simulink model "ASMod_VolEff"  (R2016b)
settings: configuration reference "CodeGenConfigSet" (kept outside this file)
values from neighbouring files (symbols this model uses):
  ASMod_facEGRCor_MAP = Calibration.Parameter    [init_ASMod_VolEff.m]    (also in init_ASMod_VolEff_SIL.m = Simulink.Parameter)
  ASMod_facEGRCor_MAPX = Calibration.Parameter    [init_ASMod_VolEff.m]    (also in init_ASMod_VolEff_SIL.m = Simulink.Parameter)
  ASMod_facEGRCor_MAPY = Calibration.Parameter    [init_ASMod_VolEff.m]    (also in init_ASMod_VolEff_SIL.m = Simulink.Parameter)
  ASMod_facIntMnfDsTempCor_C = Calibration.Parameter    [init_ASMod_VolEff.m]    (also in init_ASMod_VolEff_SIL.m = Simulink.Parameter)
  ASMod_facVolEffBas_MAP = Calibration.Parameter    [init_ASMod_VolEff.m]    (also in init_ASMod_VolEff_SIL.m = Simulink.Parameter)
  ASMod_facVolEffBas_MAPX = Calibration.Parameter    [init_ASMod_VolEff.m]    (also in init_ASMod_VolEff_SIL.m = Simulink.Parameter)
  ASMod_facVolEffBas_MAPY = Calibration.Parameter    [init_ASMod_VolEff.m]    (also in init_ASMod_VolEff_SIL.m = Simulink.Parameter)
  ASMod_nThresDwn_C = Calibration.Parameter    [init_ASMod_VolEff.m]    (also in init_ASMod_VolEff_SIL.m = Simulink.Parameter)
  ASMod_numBnk_C = Calibration.Parameter    [init_ASMod_VolEff.m]    (also in init_ASMod_VolEff_SIL.m = Simulink.Parameter)
  ASMod_tIntMnfDsRef_MAP = Calibration.Parameter    [init_ASMod_VolEff.m]    (also in init_ASMod_VolEff_SIL.m = Simulink.Parameter)
  ASMod_tIntMnfDsRef_MAPX = Calibration.Parameter    [init_ASMod_VolEff.m]    (also in init_ASMod_VolEff_SIL.m = Simulink.Parameter)
  ASMod_tIntMnfDsRef_MAPY = Calibration.Parameter    [init_ASMod_VolEff.m]    (also in init_ASMod_VolEff_SIL.m = Simulink.Parameter)
  ASMod_volEng_C = Calibration.Parameter    [init_ASMod_VolEff.m]    (also in init_ASMod_VolEff_SIL.m = Simulink.Parameter)
  Epm_numCyl_C = Calibration.Parameter    [init_ASMod_VolEff.m]
settings Model: Creator=lenovo  LastModifiedBy=zhoukai
settings ConfigSetRef: SourceLocation=Base Workspace

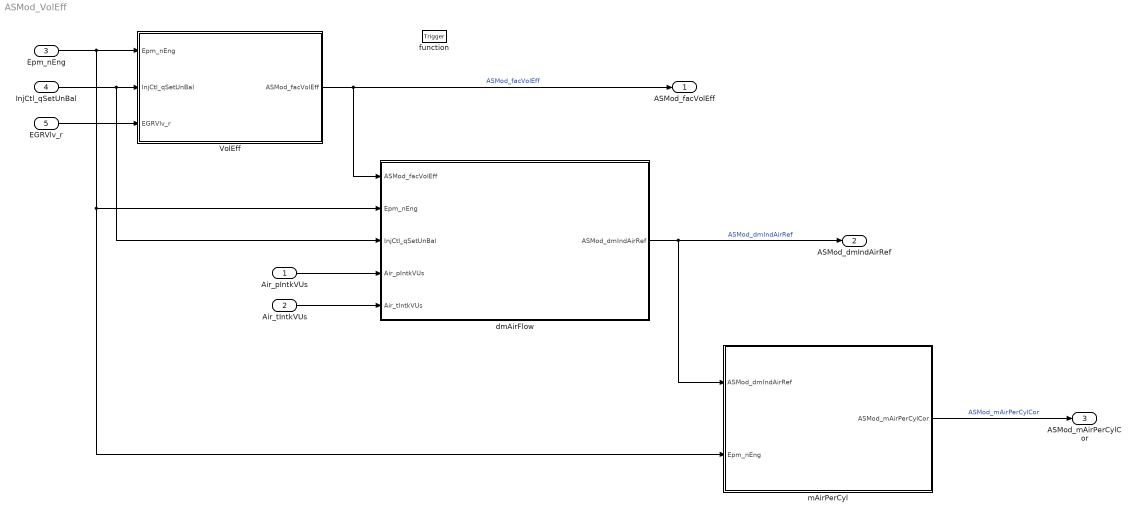
== system ASMod_VolEff ==
  Air_pIntkVUs : Inport  Tag=kPa  Description=Intake valve upstream pressure  OutMin=0  OutMax=1200  OutDataTypeStr=AirPressure_kPa
  Air_tIntkVUs : Inport  Tag=deg  Description=Intake air temperature upstream of the inlet valve  Port=2  OutMin=-200  OutMax=200  OutDataTypeStr=Temp_deg
  Epm_nEng : Inport  Tag=rpm  Description=Engine speed  Port=3  OutMin=0  OutMax=6000  OutDataTypeStr=EngSpeed_rpm
  InjCtl_qSetUnBal : Inport  Tag=mg/hub  Description=Current injection quantity  Port=4  OutMin=-319  OutMax=319  OutDataTypeStr=FuelMass_mg_hub
  EGRVlv_r : Inport  Tag=%  Description=Commanded value from application SW  Port=5  OutMin=-100  OutMax=100  OutDataTypeStr=Prc_100_rate
  function : TriggerPort  TriggerType=function-call  VariantControl=Variant
  VolEff : Subsystem
  dmAirFlow : Subsystem
  mAirPerCyl : Subsystem
  ASMod_facVolEff : Outport  Description=Volumetric efficiency of the engine  OutMin=-4  OutMax=3.9999  OutDataTypeStr=Fact8192
  ASMod_dmIndAirRef : Outport  Tag=kg/h  Description=Reference of gas mass flow into the engine while exhaust-gas recirculation is closed  Port=2  OutMin=-8192  OutMax=8191  OutDataTypeStr=AirMassPerTime
  ASMod_mAirPerCylCor : Outport  Tag=mg/hub  Description=|  Port=3  OutMin=0  OutMax=16383  OutDataTypeStr=AirMass_mg_hub
      | Dynamically corrected fresh air mass per cylinder
      | upstream of the intake manifold
  wires:
  VolEff/1(ASMod_facVolEff) -> ASMod_facVolEff/1, dmAirFlow/1(ASMod_facVolEff)  "ASMod_facVolEff"
  Air_pIntkVUs/1 -> dmAirFlow/4(Air_pIntkVUs)
  EGRVlv_r/1 -> VolEff/3(EGRVlv_r)
  dmAirFlow/1(ASMod_dmIndAirRef) -> mAirPerCyl/1(ASMod_dmIndAirRef), ASMod_dmIndAirRef/1  "ASMod_dmIndAirRef"
  InjCtl_qSetUnBal/1 -> dmAirFlow/3(InjCtl_qSetUnBal), VolEff/2(InjCtl_qSetUnBal)
  Air_tIntkVUs/1 -> dmAirFlow/5(Air_tIntkVUs)
  Epm_nEng/1 -> mAirPerCyl/2(Epm_nEng), dmAirFlow/2(Epm_nEng), VolEff/1(Epm_nEng)
  mAirPerCyl/1(ASMod_mAirPerCylCor) -> ASMod_mAirPerCylCor/1  "ASMod_mAirPerCylCor"

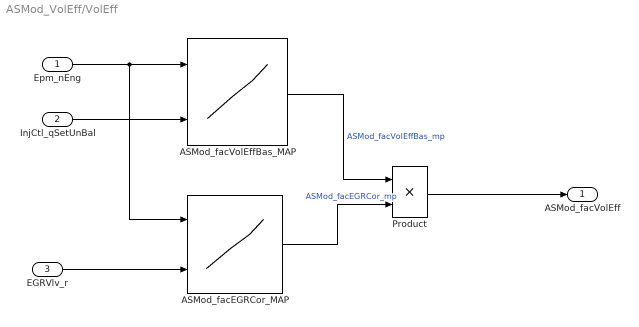
== system ASMod_VolEff/VolEff ==
  Epm_nEng : Inport
  InjCtl_qSetUnBal : Inport  Port=2
  EGRVlv_r : Inport  Port=3
  ASMod_facEGRCor_MAP : Lookup_n-D  BreakpointsForDimension1=ASMod_facEGRCor_MAPY  BreakpointsForDimension2=ASMod_facEGRCor_MAPX  BreakpointsForDimension1DataTypeStr=Inherit: Inherit from 'Breakpoint data'  BreakpointsForDimension2DataTypeStr=Inherit: Inherit from 'Breakpoint data'  Table=ASMod_facEGRCor_MAP  TableDataTypeStr=Inherit: Inherit from 'Table data'  ExtrapMethod=Clip  InternalRulePriority=Speed  OutDataTypeStr=Inherit: Inherit from 'Table data'  RndMeth=Simplest
  ASMod_facVolEffBas_MAP : Lookup_n-D  BreakpointsForDimension1=ASMod_facVolEffBas_MAPY  BreakpointsForDimension2=ASMod_facVolEffBas_MAPX  BreakpointsForDimension1DataTypeStr=Inherit: Inherit from 'Breakpoint data'  BreakpointsForDimension2DataTypeStr=Inherit: Inherit from 'Breakpoint data'  Table=ASMod_facVolEffBas_MAP  TableDataTypeStr=Inherit: Inherit from 'Table data'  ExtrapMethod=Clip  InternalRulePriority=Speed  OutDataTypeStr=Inherit: Inherit from 'Table data'  RndMeth=Simplest
  Product : Product  OutDataTypeStr=Fact8192  SaturateOnIntegerOverflow=on
  ASMod_facVolEff : Outport
  wires:
  InjCtl_qSetUnBal/1 -> ASMod_facVolEffBas_MAP/2
  Epm_nEng/1 -> ASMod_facEGRCor_MAP/1, ASMod_facVolEffBas_MAP/1
  ASMod_facVolEffBas_MAP/1 -> Product/1  "ASMod_facVolEffBas_mp"
  ASMod_facEGRCor_MAP/1 -> Product/2  "ASMod_facEGRCor_mp"
  Product/1 -> ASMod_facVolEff/1
  EGRVlv_r/1 -> ASMod_facEGRCor_MAP/2

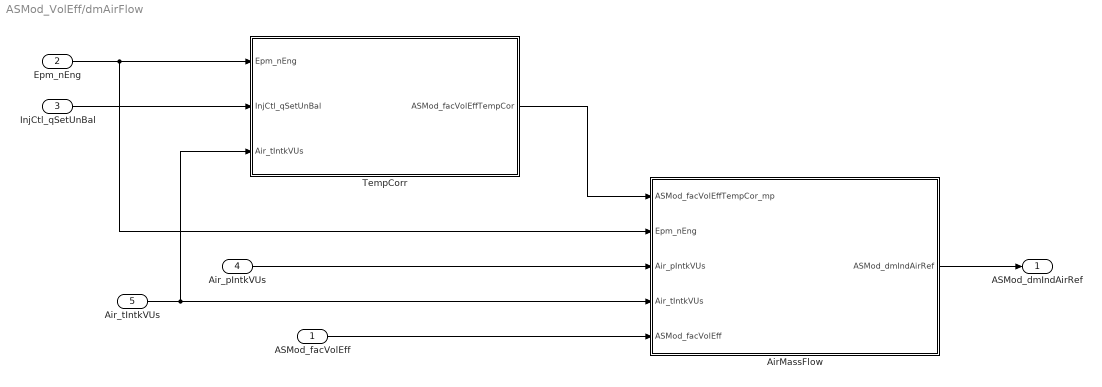
== system ASMod_VolEff/dmAirFlow ==
  ASMod_facVolEff : Inport
  Epm_nEng : Inport  Port=2
  InjCtl_qSetUnBal : Inport  Port=3
  Air_pIntkVUs : Inport  Port=4
  Air_tIntkVUs : Inport  Port=5
  AirMassFlow : Subsystem
  TempCorr : Subsystem
  ASMod_dmIndAirRef : Outport
  wires:
  InjCtl_qSetUnBal/1 -> TempCorr/2(InjCtl_qSetUnBal)
  Epm_nEng/1 -> AirMassFlow/2(Epm_nEng), TempCorr/1(Epm_nEng)
  Air_pIntkVUs/1 -> AirMassFlow/3(Air_pIntkVUs)
  Air_tIntkVUs/1 -> TempCorr/3(Air_tIntkVUs), AirMassFlow/4(Air_tIntkVUs)
  TempCorr/1(ASMod_facVolEffTempCor) -> AirMassFlow/1(ASMod_facVolEffTempCor_mp)
  AirMassFlow/1(ASMod_dmIndAirRef) -> ASMod_dmIndAirRef/1
  ASMod_facVolEff/1 -> AirMassFlow/5(ASMod_facVolEff)

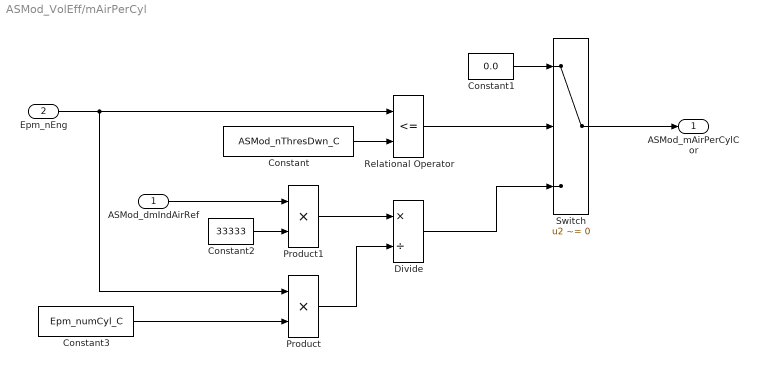
== system ASMod_VolEff/mAirPerCyl ==
  ASMod_dmIndAirRef : Inport  Description=Real number of cylinder  OutMin=-8192  OutMax=8191  OutDataTypeStr=AirMassPerTime
  Epm_nEng : Inport  Tag=rpm  Description=Engine speed  Port=2  OutMin=0  OutMax=6000  OutDataTypeStr=EngSpeed_rpm
  Constant : Constant  Value=ASMod_nThresDwn_C
  Constant1 : Constant  Value=0.0  OutDataTypeStr=Inherit: Inherit via back propagation
  Constant2 : Constant  Value=33333  OutDataTypeStr=fixdt(1,16)
  Constant3 : Constant  Value=Epm_numCyl_C
  Divide : Product  Inputs=*/  OutDataTypeStr=Inherit: Inherit via back propagation  SaturateOnIntegerOverflow=on
  Product : Product  SaturateOnIntegerOverflow=on
  Product1 : Product  SaturateOnIntegerOverflow=on
  Relational Operator : RelationalOperator  Operator=<=  OutDataTypeStr=boolean  RndMeth=Simplest  InputSameDT=on
  Switch : Switch  Criteria=u2 ~= 0  SaturateOnIntegerOverflow=on  InputSameDT=on
  ASMod_mAirPerCylCor : Outport  Tag=mg/hub  Description=|  OutMin=0  OutMax=16383  OutDataTypeStr=AirMass_mg_hub
      | Dynamically corrected fresh air mass per cylinder
      | upstream of the intake manifold
  wires:
  Epm_nEng/1 -> Product/1, Relational Operator/1
  Constant/1 -> Relational Operator/2
  Relational Operator/1 -> Switch/2
  Constant1/1 -> Switch/1
  Constant3/1 -> Product/2
  ASMod_dmIndAirRef/1 -> Product1/1
  Constant2/1 -> Product1/2
  Product1/1 -> Divide/1
  Product/1 -> Divide/2
  Divide/1 -> Switch/3
  Switch/1 -> ASMod_mAirPerCylCor/1

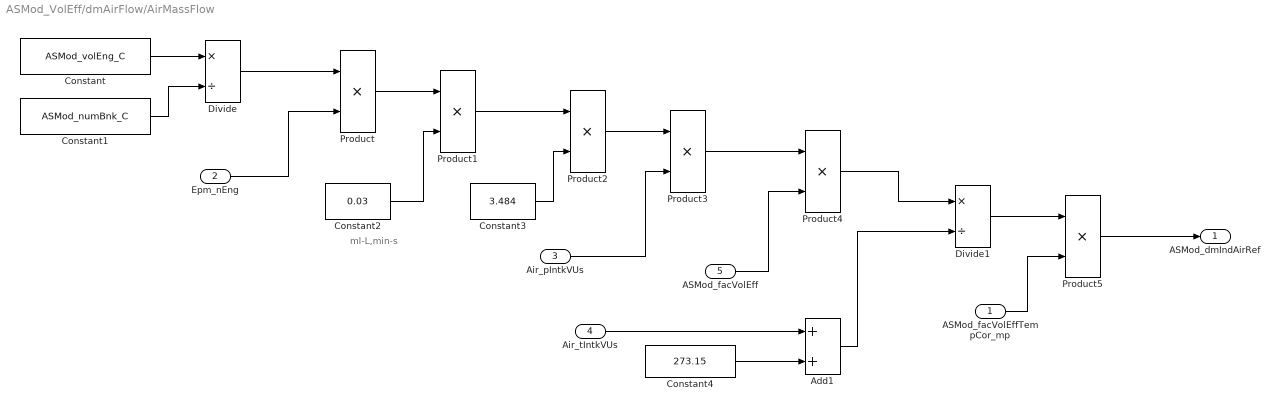
== system ASMod_VolEff/dmAirFlow/AirMassFlow ==
  note: ml-L,min-s
  ASMod_facVolEffTempCor_mp : Inport
  Epm_nEng : Inport  Port=2
  Air_pIntkVUs : Inport  Port=3
  Air_tIntkVUs : Inport  Port=4
  ASMod_facVolEff : Inport  Port=5
  Add1 : Sum  AccumDataTypeStr=Temp_deg  OutDataTypeStr=TempDiff_Kelv
  Constant : Constant  Value=ASMod_volEng_C
  Constant1 : Constant  Value=ASMod_numBnk_C
  Constant2 : Constant  Value=0.03  OutDataTypeStr=fixdt(1,16,10)
  Constant3 : Constant  Value=3.484  OutDataTypeStr=fixdt(0,16,10)
  Constant4 : Constant  Value=273.15  OutDataTypeStr=Temp_deg
  Divide : Product  Inputs=*/  OutDataTypeStr=fixdt(0,16,10)  SaturateOnIntegerOverflow=on
  Divide1 : Product  Inputs=*/  OutDataTypeStr=Inherit: Same as first input
  Product : Product  OutDataTypeStr=fixdt(0,32,10)  SaturateOnIntegerOverflow=on
  Product1 : Product  OutDataTypeStr=Inherit: Same as first input
  Product2 : Product  OutDataTypeStr=Inherit: Same as first input
  Product3 : Product  SaturateOnIntegerOverflow=on  OutDataTypeStr=Inherit: Same as first input
  Product4 : Product  SaturateOnIntegerOverflow=on  OutDataTypeStr=Inherit: Same as first input
  Product5 : Product  OutDataTypeStr=Inherit: Inherit via back propagation
  ASMod_dmIndAirRef : Outport
  wires:
  Constant1/1 -> Divide/2
  ASMod_facVolEffTempCor_mp/1 -> Product5/2
  Divide1/1 -> Product5/1
  Product1/1 -> Product2/1
  Product5/1 -> ASMod_dmIndAirRef/1
  Epm_nEng/1 -> Product/2
  Product/1 -> Product1/1
  Constant2/1 -> Product1/2
  Constant3/1 -> Product2/2
  Product2/1 -> Product3/1
  Air_pIntkVUs/1 -> Product3/2
  Constant/1 -> Divide/1
  Divide/1 -> Product/1
  Product3/1 -> Product4/1
  ASMod_facVolEff/1 -> Product4/2
  Product4/1 -> Divide1/1
  Add1/1 -> Divide1/2
  Air_tIntkVUs/1 -> Add1/1
  Constant4/1 -> Add1/2

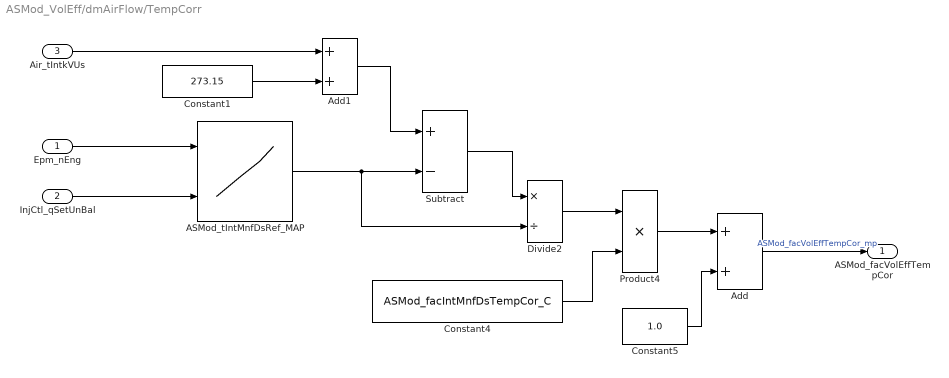
== system ASMod_VolEff/dmAirFlow/TempCorr ==
  Epm_nEng : Inport
  InjCtl_qSetUnBal : Inport  Port=2
  Air_tIntkVUs : Inport  Port=3
  ASMod_tIntMnfDsRef_MAP : Lookup_n-D  BreakpointsForDimension1=ASMod_tIntMnfDsRef_MAPY  BreakpointsForDimension2=ASMod_tIntMnfDsRef_MAPX  BreakpointsForDimension1DataTypeStr=Inherit: Inherit from 'Breakpoint data'  BreakpointsForDimension2DataTypeStr=Inherit: Inherit from 'Breakpoint data'  Table=ASMod_tIntMnfDsRef_MAP  TableDataTypeStr=Inherit: Inherit from 'Table data'  ExtrapMethod=Clip  InternalRulePriority=Speed  OutDataTypeStr=Inherit: Inherit from 'Table data'  RndMeth=Simplest
  Add : Sum  SaturateOnIntegerOverflow=on
  Add1 : Sum  AccumDataTypeStr=Temp_deg  OutDataTypeStr=TempDiff_Kelv
  Constant1 : Constant  Value=273.15  OutDataTypeStr=Temp_deg
  Constant4 : Constant  Value=ASMod_facIntMnfDsTempCor_C
  Constant5 : Constant  Value=1.0  OutDataTypeStr=Fact8192
  Divide2 : Product  Inputs=*/  OutDataTypeStr=Fact8192  SaturateOnIntegerOverflow=on
  Product4 : Product  OutDataTypeStr=Fact8192  SaturateOnIntegerOverflow=on
  Subtract : Sum  Inputs=+-  SaturateOnIntegerOverflow=on
  ASMod_facVolEffTempCor : Outport
  wires:
  Add/1 -> ASMod_facVolEffTempCor/1  "ASMod_facVolEffTempCor_mp"
  Product4/1 -> Add/1
  Constant5/1 -> Add/2
  InjCtl_qSetUnBal/1 -> ASMod_tIntMnfDsRef_MAP/2
  ASMod_tIntMnfDsRef_MAP/1 -> Divide2/2, Subtract/2
  Constant4/1 -> Product4/2
  Divide2/1 -> Product4/1
  Subtract/1 -> Divide2/1
  Air_tIntkVUs/1 -> Add1/1
  Epm_nEng/1 -> ASMod_tIntMnfDsRef_MAP/1
  Add1/1 -> Subtract/1
  Constant1/1 -> Add1/2
